simulink model "xz2dof_traj"  (R2023a)
settings: Solver=ode4  StartTime=0.0  StopTime=50  FixedStep=0.0001  RelTol=1e-3
values from neighbouring files (symbols this model uses):
  B1 = inv(B)    [grasp_test.m]    (also in my_mpc.m = inv(B0); xz2dof_para.m)
  C1 = C    [grasp_test.m]    (also in xz2dof_para.m)
  g = 9.8    [grasp_test.m]    (also in my_mpc.m; track_test.m; xz2dof_para.m)
  hL1 = 0.001    [grasp_test.m]    (also in my_mpc.m; xz2dof_para.m)
  hL2 = 0.001    [grasp_test.m]    (also in my_mpc.m; xz2dof_para.m)
  Iyy = 3*0.114    (= 0.342)    [my_mpc.m]    (also in track_test.m; xz2dof_para.m)
  kdq1 = 800    [grasp_test.m]    (also in xz2dof_para.m)
  kdq2 = 300    [grasp_test.m]    (also in xz2dof_para.m)
  kdx = 0.8    [track_test.m]    (also in xz2dof_para.m = 17)
  kdz = 1.5    [track_test.m]    (also in xz2dof_para.m = 50)
  kiq1 = 500    [grasp_test.m]    (also in xz2dof_para.m)
  kiq2 = 1000    [grasp_test.m]    (also in xz2dof_para.m)
  kix = 0    [track_test.m]    (also in xz2dof_para.m = 10)
  kiz = 0    [track_test.m]    (also in xz2dof_para.m)
  kpq1 = 1200    [grasp_test.m]    (also in xz2dof_para.m)
  kpq2 = 2000    [grasp_test.m]    (also in xz2dof_para.m)
  kpx = 1    [track_test.m]    (also in xz2dof_para.m = 180)
  kpz = 1.8    [track_test.m]    (also in xz2dof_para.m = 50)
  ktd = 10    [grasp_test.m]    (also in xz2dof_para.m)
  ktp = 1    [grasp_test.m]    (also in xz2dof_para.m)
  L1 = 0.12    [grasp_test.m]    (also in my_mpc.m; xz2dof_para.m)
  L2 = 0.12    [grasp_test.m]    (also in my_mpc.m; xz2dof_para.m)
  mb = 1.58    [my_mpc.m]    (also in track_test.m = 1.8; xz2dof_para.m = 1.8)
  mL1 = 0.1    [my_mpc.m]    (also in track_test.m = 0.08; xz2dof_para.m = 0.08)
  mL2 = 0.1    [my_mpc.m]    (also in track_test.m = 0.08; xz2dof_para.m = 0.08)
  ms = mb+mL1+mL2    (= 1.78)    [my_mpc.m]    (also in track_test.m = 1.96; xz2dof_para.m = 1.96)
  q1 = pi/2    (= 1.57079632679)    [grasp_test.m]    (also in my_mpc.m = xd(4) + xe(4); xz2dof_para.m)
  q2 = 0    [grasp_test.m]    (also in my_mpc.m = xd(5) + xe(5); xz2dof_para.m)
  step_num = T/tstep    (= 100)    [grasp_test.m]
undefined symbols (not defined in the file or in its folder): arm_traj
libraries: dspindex x1
settings Model: Creator=Administrator  LastModifiedBy=User
settings SolverCC: AlgebraicLoopSolver=TrustRegion
settings DataIOCC: ReturnWorkspaceOutputs=off
settings DebuggingCC: UnconnectedInputMsg=warning  UnconnectedOutputMsg=warning  UnconnectedLineMsg=warning
settings ModelReferenceCC: EnableRefExpFcnMdlSchedulingChecks=on
settings SFSimCC: CustomCodeUndefinedFunction=UseInterfaceOnly

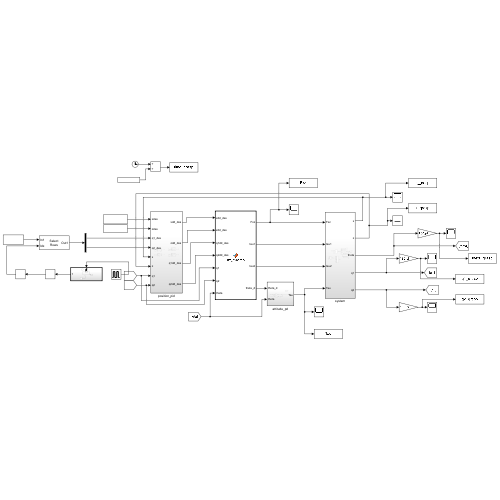
[thumbnail: Simulink's stored preview of the top-level diagram]
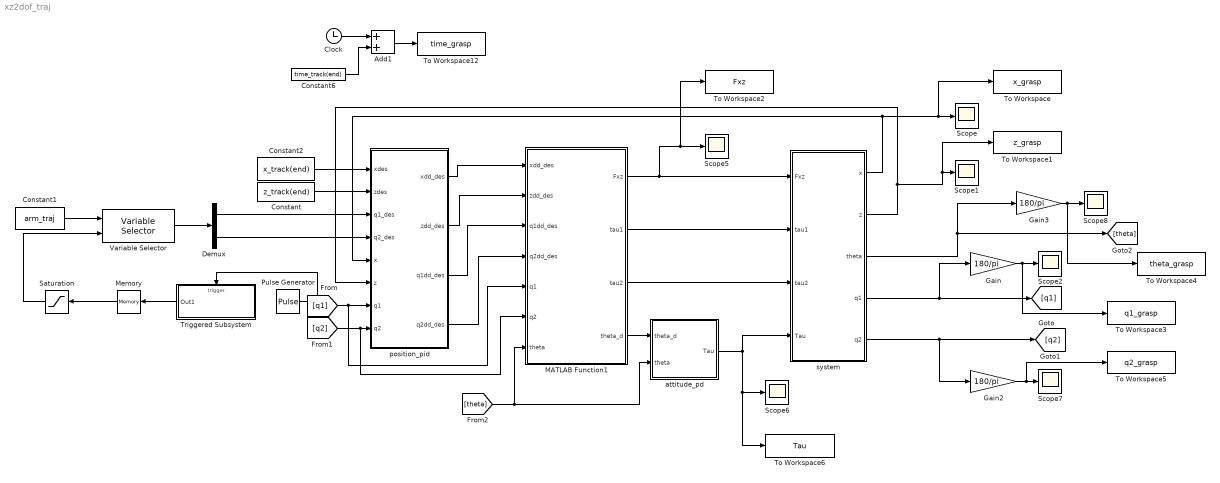
== system xz2dof_traj ==
  Add1 : Sum
  Clock : Clock
  Constant : Constant  Value=z_track(end)
  Constant1 : Constant  Value=arm_traj
  Constant2 : Constant  Value=x_track(end)
  Constant6 : Constant  Value=time_track(end)
  Demux : Demux  Outputs=2
  Gain : Gain  Gain=180/pi
  Gain2 : Gain  Gain=180/pi
  Gain3 : Gain  Gain=180/pi
  MATLAB Function1 : MATLAB Function  TreatAsAtomicUnit=on
  Memory : Memory
  Pulse Generator : DiscretePulseGenerator  PulseType=Time based  Period=0.5  PulseWidth=50
  Saturation : Saturate  UpperLimit=step_num  LowerLimit=0
  Scope{,1..2,5..8} (7 alike) : Scope
  To Workspace : ToWorkspace  VariableName=x_grasp  SampleTime=-1
  To Workspace1 : ToWorkspace  VariableName=z_grasp  SampleTime=-1
  To Workspace12 : ToWorkspace  VariableName=time_grasp  SampleTime=-1
  To Workspace2 : ToWorkspace  VariableName=Fxz  SampleTime=-1
  To Workspace3 : ToWorkspace  VariableName=q1_grasp  SampleTime=-1
  To Workspace4 : ToWorkspace  VariableName=theta_grasp  SampleTime=-1
  To Workspace5 : ToWorkspace  VariableName=q2_grasp  SampleTime=-1
  To Workspace6 : ToWorkspace  VariableName=Tau  SampleTime=-1
  Triggered Subsystem : Subsystem  TreatAsAtomicUnit=on
  Variable Selector : dspindex/Variable Selector  NumInputs=1  rowsOrCols=Rows  IdxMode=Variable  Elements=[1 3]  ZerOneIdxMode=Zero-based  errmode=Clip Index  FillMode=on  FillValues=0
  attitude_pd : Subsystem
  position_pid : Subsystem
  system : Subsystem
  wires:
  MATLAB Function1/4(theta_d) -> attitude_pd/1(theta_d)
  MATLAB Function1/1(Fxz) -> To Workspace2/1, Scope5/1, system/1(Fxz)
  attitude_pd/1(Tau) -> To Workspace6/1, Scope6/1, system/4(Tau)
  system/2(z) -> To Workspace1/1, Scope1/1, position_pid/6(z)
  system/1(x) -> To Workspace/1, Scope/1, position_pid/5(x)
  Gain/1 -> To Workspace3/1, Scope2/1
  Constant/1 -> position_pid/2(zdes)
  Constant2/1 -> position_pid/1(xdes)
  Add1/1 -> To Workspace12/1
  Clock/1 -> Add1/1
  Constant6/1 -> Add1/2
  [q1] -> MATLAB Function1/5(q1), position_pid/7(q1)
  system/5(q2) -> Gain2/1, [q2]
  Gain2/1 -> To Workspace5/1, Scope7/1
  [q2] -> MATLAB Function1/6(q2), position_pid/8(q2)
  position_pid/1(xdd_des) -> MATLAB Function1/1(xdd_des)
  position_pid/2(zdd_des) -> MATLAB Function1/2(zdd_des)
  position_pid/3(q1dd_des) -> MATLAB Function1/3(q1dd_des)
  position_pid/4(q2dd_des) -> MATLAB Function1/4(q2dd_des)
  MATLAB Function1/2(tau1) -> system/2(tau1)
  MATLAB Function1/3(tau2) -> system/3(tau2)
  Gain3/1 -> To Workspace4/1, Scope8/1
  system/3(theta) -> [theta], Gain3/1
  [theta] -> attitude_pd/2(theta), MATLAB Function1/7(theta)
  system/4(q1) -> Gain/1, [q1]
  Constant1/1 -> Variable Selector/1
  Variable Selector/1 -> Demux/1
  Memory/1 -> Saturation/1
  Triggered Subsystem/1(Out1) -> Memory/1
  Pulse Generator/1 -> Triggered Subsystem/Trigger
  Saturation/1 -> Variable Selector/2
  Demux/1 -> position_pid/3(q1_des)
  Demux/2 -> position_pid/4(q2_des)

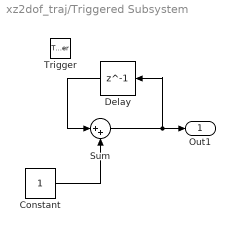
== system xz2dof_traj/Triggered Subsystem ==
  Trigger : TriggerPort  VariantControl=Variant
  Constant : Constant
  Delay : Delay  DelayLength=1
  Sum : Sum  Inputs=|++
  Out1 : Outport  VectorParamsAs1DForOutWhenUnconnected=off
  wires:
  Sum/1 -> Delay/1, Out1/1
  Constant/1 -> Sum/2
  Delay/1 -> Sum/1

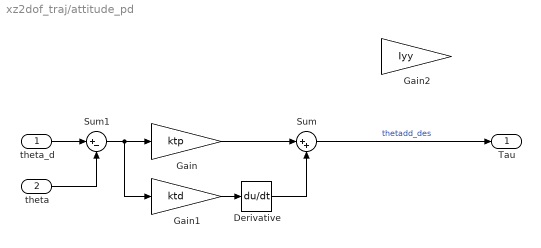
== system xz2dof_traj/attitude_pd ==
  theta_d : Inport
  theta : Inport  Port=2
  Derivative : Derivative
  Gain : Gain  Gain=ktp
  Gain1 : Gain  Gain=ktd
  Gain2 : Gain  Gain=Iyy
  Sum : Sum  Inputs=|++
  Sum1 : Sum  Inputs=|+-
  Tau : Outport  VectorParamsAs1DForOutWhenUnconnected=off
  wires:
  theta/1 -> Sum1/2
  Gain1/1 -> Derivative/1
  Derivative/1 -> Sum/2
  Sum1/1 -> Gain1/1, Gain/1
  Gain/1 -> Sum/1
  theta_d/1 -> Sum1/1
  Sum/1 -> Tau/1  "thetadd_des"

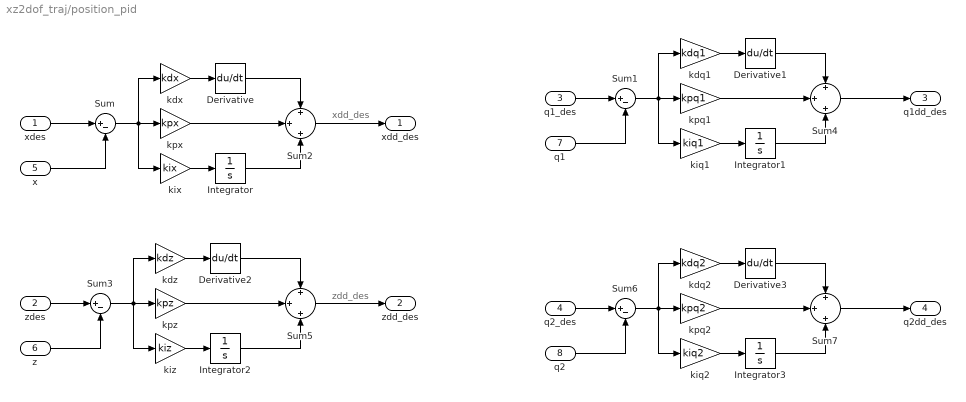
== system xz2dof_traj/position_pid ==
  note: zdd_des
  note: xdd_des
  xdes : Inport
  zdes : Inport  Port=2
  q1_des : Inport  Port=3
  q2_des : Inport  Port=4
  x : Inport  Port=5
  z : Inport  Port=6
  q1 : Inport  Port=7
  q2 : Inport  Port=8
  Derivative{,1..3} (4 alike) : Derivative
  Integrator{,1..3} (4 alike) : Integrator
  Sum{,1,3,6} (4 alike) : Sum  Inputs=|+-
  Sum{2,4..5,7} (4 alike) : Sum  Inputs=+|+|+
  kdq1 : Gain  Gain=kdq1
  kdq2 : Gain  Gain=kdq2
  kdx : Gain  Gain=kdx
  kdz : Gain  Gain=kdz
  kiq1 : Gain  Gain=kiq1
  kiq2 : Gain  Gain=kiq2
  kix : Gain  Gain=kix
  kiz : Gain  Gain=kiz
  kpq1 : Gain  Gain=kpq1
  kpq2 : Gain  Gain=kpq2
  kpx : Gain  Gain=kpx
  kpz : Gain  Gain=kpz
  xdd_des : Outport  VectorParamsAs1DForOutWhenUnconnected=off
  zdd_des : Outport  Port=2  VectorParamsAs1DForOutWhenUnconnected=off
  q1dd_des : Outport  Port=3  VectorParamsAs1DForOutWhenUnconnected=off
  q2dd_des : Outport  Port=4  VectorParamsAs1DForOutWhenUnconnected=off
  wires:
  kpz/1 -> Sum5/2
  kiz/1 -> Integrator2/1
  xdes/1 -> Sum/1
  kpx/1 -> Sum2/2
  z/1 -> Sum3/2
  Sum/1 -> kix/1, kpx/1, kdx/1
  kdx/1 -> Derivative/1
  Integrator/1 -> Sum2/3
  kdz/1 -> Derivative2/1
  Derivative/1 -> Sum2/1
  Derivative2/1 -> Sum5/1
  Sum3/1 -> kiz/1, kpz/1, kdz/1
  Integrator2/1 -> Sum5/3
  kix/1 -> Integrator/1
  x/1 -> Sum/2
  zdes/1 -> Sum3/1
  kpq1/1 -> Sum4/2
  kiq1/1 -> Integrator1/1
  Integrator1/1 -> Sum4/3
  kdq1/1 -> Derivative1/1
  Derivative1/1 -> Sum4/1
  Sum1/1 -> kiq1/1, kpq1/1, kdq1/1
  q1/1 -> Sum1/2
  q1_des/1 -> Sum1/1
  Sum2/1 -> xdd_des/1
  Sum5/1 -> zdd_des/1
  Sum4/1 -> q1dd_des/1
  Sum7/1 -> q2dd_des/1
  q2_des/1 -> Sum6/1
  Sum6/1 -> kiq2/1, kpq2/1, kdq2/1
  Derivative3/1 -> Sum7/1
  q2/1 -> Sum6/2
  kdq2/1 -> Derivative3/1
  Integrator3/1 -> Sum7/3
  kiq2/1 -> Integrator3/1
  kpq2/1 -> Sum7/2

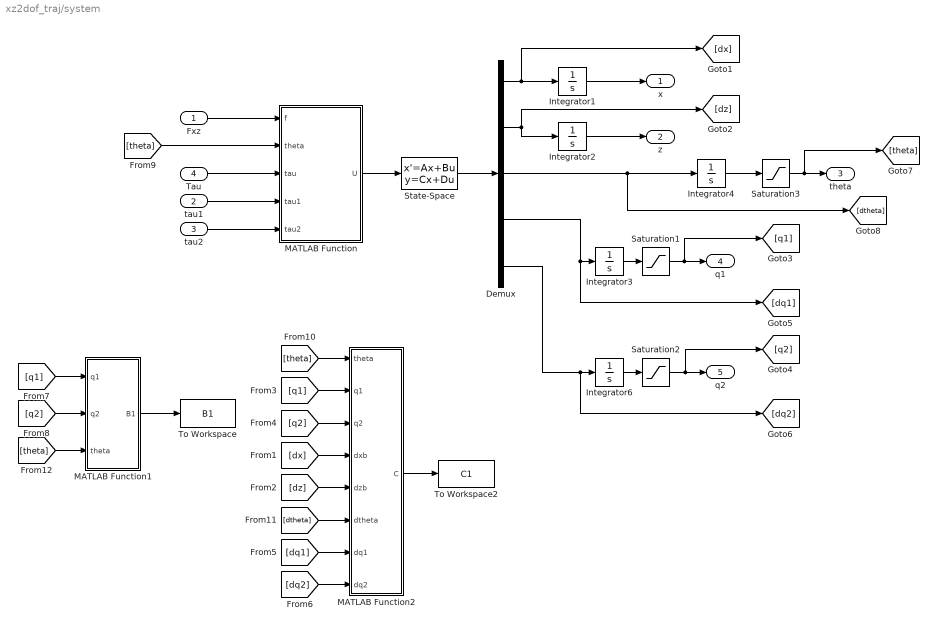
== system xz2dof_traj/system ==
  Fxz : Inport
  tau1 : Inport  Port=2
  tau2 : Inport  Port=3
  Tau : Inport  Port=4
  Demux : Demux  Outputs=5
  Integrator1 : Integrator  InitialCondition=x_track(end)
  Integrator2 : Integrator  InitialCondition=z_track(end)
  Integrator3 : Integrator  InitialCondition=pi/2
  Integrator4 : Integrator
  Integrator6 : Integrator
  MATLAB Function : MATLAB Function  TreatAsAtomicUnit=on
  MATLAB Function1 : MATLAB Function  TreatAsAtomicUnit=on
  MATLAB Function2 : MATLAB Function  TreatAsAtomicUnit=on
  Saturation1 : Saturate  UpperLimit=pi  LowerLimit=-pi
  Saturation2 : Saturate  UpperLimit=pi  LowerLimit=-pi
  Saturation3 : Saturate  UpperLimit=pi/2  LowerLimit=-pi/2
  State-Space : StateSpace  A=-B1*C1  B=B1  C=[1 0 0 0 0;0 1 0 0 0;0 0 1 0 0;0 0 0 1 0;0 0 0 0 1]  D=[0 0 0 0 0;0 0 0 0 0;0 0 0 0 0;0 0 0 0 0;0 0 0 0 0]  InitialCondition=0
  To Workspace : ToWorkspace  VariableName=B1  SaveFormat=Timeseries  SampleTime=-1
  To Workspace2 : ToWorkspace  VariableName=C1  SaveFormat=Timeseries  SampleTime=-1
  x : Outport  VectorParamsAs1DForOutWhenUnconnected=off
  z : Outport  Port=2  VectorParamsAs1DForOutWhenUnconnected=off
  theta : Outport  Port=3  VectorParamsAs1DForOutWhenUnconnected=off
  q1 : Outport  Port=4  VectorParamsAs1DForOutWhenUnconnected=off
  q2 : Outport  Port=5  VectorParamsAs1DForOutWhenUnconnected=off
  wires:
  Fxz/1 -> MATLAB Function/1(f)
  tau1/1 -> MATLAB Function/4(tau1)
  MATLAB Function/1(U) -> State-Space/1
  MATLAB Function1/1(B1) -> To Workspace/1
  State-Space/1 -> Demux/1
  Demux/1 -> [dx], Integrator1/1
  Demux/2 -> [dz], Integrator2/1
  Integrator1/1 -> x/1
  Integrator2/1 -> z/1
  Integrator3/1 -> Saturation1/1
  Demux/4 -> [dq1], Integrator3/1
  Saturation1/1 -> [q1], q1/1
  Saturation2/1 -> q2/1, [q2]
  Integrator6/1 -> Saturation2/1
  Demux/5 -> Integrator6/1, [dq2]
  [dx] -> MATLAB Function2/4(dxb)
  [dz] -> MATLAB Function2/5(dzb)
  [q1] -> MATLAB Function2/2(q1)
  [q2] -> MATLAB Function2/3(q2)
  [dq1] -> MATLAB Function2/7(dq1)
  [dq2] -> MATLAB Function2/8(dq2)
  [q1] -> MATLAB Function1/1(q1)
  [q2] -> MATLAB Function1/2(q2)
  [theta] -> MATLAB Function/2(theta)
  [theta] -> MATLAB Function2/1(theta)
  [dtheta] -> MATLAB Function2/6(dtheta)
  [theta] -> MATLAB Function1/3(theta)
  tau2/1 -> MATLAB Function/5(tau2)
  Tau/1 -> MATLAB Function/3(tau)
  Saturation3/1 -> [theta], theta/1
  Integrator4/1 -> Saturation3/1
  Demux/3 -> [dtheta], Integrator4/1
  MATLAB Function2/1(C) -> To Workspace2/1

== matlab function xz2dof_traj/system/MATLAB Function1 ==
  data: q1 input; q2 input; theta input; B1 output; mL1 parameter; mL2 parameter; mb parameter; L1 parameter; L2 parameter; hL1 parameter; hL2 parameter; Iyy parameter
function B1 = Bout(q1, q2, theta, mL1, mL2, mb, L1, L2, hL1, hL2, Iyy)
B = zeros(5,5);

B(1,1) = mL1 + mL2 + mb; B(1,2) = 0;
B(1,3) = (mL1*L1/2 + mL2*L1)*sin(q1-theta) + (mL2*L2/2)*sin(q1+q2-theta);
B(1,4) = -(mL1*L1/2 + mL2*L1)*sin(q1-theta) - (mL2*L2/2)*sin(q1+q2-theta);
B(1,5) = -(mL2*L2/2)*sin(q1+q2-theta);

B(2,1) = 0; B(2,2) = mL1 + mL2 + mb;
B(2,3) = -(mL1*L1/2 + mL2*L1)*cos(q1-theta) - (mL2*L2/2)*cos(q1+q2-theta);
B(2,4) = (mL1*L1/2 + mL2*L1)*cos(q1-theta) + (mL2*L2/2)*cos(q1+q2-theta);
B(2,5) = (mL2*L2/2)*cos(q1+q2-theta);

B(3,1) = (mL1*L1/2 + mL2*L1)*sin(q1-theta) + (mL2*L2/2)*sin(q1+q2-theta);
B(3,2) = -(mL1*L1/2 + mL2*L1)*cos(q1-theta) - (mL2*L2/2)*cos(q1+q2-theta);
B(3,3) = hL1 + hL2 + Iyy + mL1*(L1/2)^2 + mL2*(L1^2 + (L2/2)^2 + L1*L2*cos(q2)); 
B(3,4) = -mL2*(L1^2 + (L2/2)^2 + L1*L2*cos(q2)) - mL1*(L1/2)^2;
B(3,5) = -mL2*L2/2*(L2/2+L1*cos(q2));

B(4,1) = -(mL1*L1/2 + mL2*L1)*sin(q1-theta) - (mL2*L2/2)*sin(q1+q2-theta);
B(4,2) = (mL1*L1/2 + mL2*L1)*cos(q1-theta) + (mL2*L2/2)*cos(q1+q2-theta);
B(4,3) = -mL2*(L1^2 + (L2/2)^2 + L1*L2*cos(q2)) - mL1*(L1/2)^2;
B(4,4) = mL1*(L1/2)^2 + mL2*(L1^2 + (L2/2)^2 + L1*L2*cos(q2));
B(4,5) = mL2*L2/2*(L1*cos(q2) + L2/2);

B(5,1) = -(mL2*L2/2)*sin(q1+q2-theta);
B(5,2) = (mL2*L2/2)*cos(q1+q2-theta);
B(5,3) = -mL2*L2/2*(L2/2+L1*cos(q2));
B(5,4) = mL2*L2/2*(L1*cos(q2) + L2/2);
B(5,5) = mL2*L2*L2/4;

B1 = inv(B);

end

== matlab function xz2dof_traj/system/MATLAB Function ==
  data: f input; theta input; tau input; tau1 input; U output; tau2 input; q1 parameter; q2 parameter; g parameter; mL1 parameter; mL2 parameter; mb parameter; L1 parameter; L2 parameter
function U = Uout(f,theta,tau,tau1,tau2,q1,q2,g, mL1, mL2, mb, L1, L2)
u = zeros(5,1);
G = zeros(5,1);
U = zeros(5,1);

% f = f1+f2+f3+f4 是总升力
% tau是俯仰力矩
% tau1,tau2是关节力矩
u(1,1) = f*sin(theta);
u(2,1) = f*cos(theta);
u(3,1) = tau;
u(4,1) = tau1;
u(5,1) = tau2;

%% 计算G
G(1,1) = 0;
G(2,1) = (mL1 + mL2 + mb)*g;
G(3,1) = - g*mL1*(L1/2*cos(q1-theta)) - g*mL2*(L1*cos(q1-theta)+L2/2*cos(q1+q2-theta));
G(4,1) = g*mL1*(L1/2*cos(q1-theta)) + g*mL2*(L1*cos(q1-theta)+L2/2*cos(q1+q2-theta));
G(5,1) = g*mL2*L2/2*cos(q1 + q2-theta);

U = u - G;
end

== matlab function xz2dof_traj/system/MATLAB Function2 ==
  data: theta input; C output; q1 input; q2 input; dxb input; dzb input; dtheta input; dq1 input; dq2 input; mL1 parameter; mL2 parameter; L1 parameter; L2 parameter
function C = Cout(theta, q1, q2, dxb, dzb, dtheta, dq1, dq2, mL1, mL2, L1, L2)
C = zeros(5,5);

C(1,1) = 0; C(1,2) = 0;
C(1,3) =  dq1*(cos(q1 - theta)*((L1*mL1)/2 + L1*mL2) + (L2*mL2*cos(q1 + q2 - theta))/2) - dtheta*(cos(q1 - theta)*((L1*mL1)/2 + L1*mL2) + (L2*mL2*cos(q1 + q2 - theta))/2) + (L2*dq2*mL2*cos(q1 + q2 - theta))/2;
C(1,4) = dtheta*(cos(q1 - theta)*((L1*mL1)/2 + L1*mL2) + (L2*mL2*cos(q1 + q2 - theta))/2) - dq1*(cos(q1 - theta)*((L1*mL1)/2 + L1*mL2) + (L2*mL2*cos(q1 + q2 - theta))/2) - (L2*dq2*mL2*cos(q1 + q2 - theta))/2;
C(1,5) = (L2*dtheta*mL2*cos(q1 + q2 - theta))/2 - (L2*dq2*mL2*cos(q1 + q2 - theta))/2 - (L2*dq1*mL2*cos(q1 + q2 - theta))/2;

C(2,1) = 0; C(2,2) = 0;
C(2,3) = dq1*(sin(q1 - theta)*((L1*mL1)/2 + L1*mL2) + (L2*mL2*sin(q1 + q2 - theta))/2) - dtheta*(sin(q1 - theta)*((L1*mL1)/2 + L1*mL2) + (L2*mL2*sin(q1 + q2 - theta))/2) + (L2*dq2*mL2*sin(q1 + q2 - theta))/2;
C(2,4) = dtheta*(sin(q1 - theta)*((L1*mL1)/2 + L1*mL2) + (L2*mL2*sin(q1 + q2 - theta))/2) - dq1*(sin(q1 - theta)*((L1*mL1)/2 + L1*mL2) + (L2*mL2*sin(q1 + q2 - theta))/2) - (L2*dq2*mL2*sin(q1 + q2 - theta))/2;
C(2,5) = (L2*dtheta*mL2*sin(q1 + q2 - theta))/2 - (L2*dq2*mL2*sin(q1 + q2 - theta))/2 - (L2*dq1*mL2*sin(q1 + q2 - theta))/2;
 
C(3,1) = dq1*(cos(q1 - theta)*((L1*mL1)/2 + L1*mL2) + (L2*mL2*cos(q1 + q2 - theta))/2) - dtheta*(cos(q1 - theta)*((L1*mL1)/2 + L1*mL2) + (L2*mL2*cos(q1 + q2 - theta))/2) + (L2*dq2*mL2*cos(q1 + q2 - theta))/2;
C(3,2) = dq1*(sin(q1 - theta)*((L1*mL1)/2 + L1*mL2) + (L2*mL2*sin(q1 + q2 - theta))/2) - dtheta*(sin(q1 - theta)*((L1*mL1)/2 + L1*mL2) + (L2*mL2*sin(q1 + q2 - theta))/2) + (L2*dq2*mL2*sin(q1 + q2 - theta))/2;
C(3,3) = - dxb*(cos(q1 - theta)*((L1*mL1)/2 + L1*mL2) + (L2*mL2*cos(q1 + q2 - theta))/2) - dzb*(sin(q1 - theta)*((L1*mL1)/2 + L1*mL2) + (L2*mL2*sin(q1 + q2 - theta))/2) - (L1*L2*dq2*mL2*sin(q2))/2;
C(3,4) = dxb*(cos(q1 - theta)*((L1*mL1)/2 + L1*mL2) + (L2*mL2*cos(q1 + q2 - theta))/2) + dzb*(sin(q1 - theta)*((L1*mL1)/2 + L1*mL2) + (L2*mL2*sin(q1 + q2 - theta))/2) + (L1*L2*dq2*mL2*sin(q2))/2;
C(3,5) = (L2*dzb*mL2*sin(q1 + q2 - theta))/2 + (L2*dxb*mL2*cos(q1 + q2 - theta))/2 + (L1*L2*dq1*mL2*sin(q2))/2 + (L1*L2*dq2*mL2*sin(q2))/2 - (L1*L2*dtheta*mL2*sin(q2))/2;

C(4,1) = dtheta*(cos(q1 - theta)*((L1*mL1)/2 + L1*mL2) + (L2*mL2*cos(q1 + q2 - theta))/2) - dq1*(cos(q1 - theta)*((L1*mL1)/2 + L1*mL2) + (L2*mL2*cos(q1 + q2 - theta))/2) - (L2*dq2*mL2*cos(q1 + q2 - theta))/2;
C(4,2) = dtheta*(sin(q1 - theta)*((L1*mL1)/2 + L1*mL2) + (L2*mL2*sin(q1 + q2 - theta))/2) - dq1*(sin(q1 - theta)*((L1*mL1)/2 + L1*mL2) + (L2*mL2*sin(q1 + q2 - theta))/2) - (L2*dq2*mL2*sin(q1 + q2 - theta))/2;
C(4,3) = dxb*(cos(q1 - theta)*((L1*mL1)/2 + L1*mL2) + (L2*mL2*cos(q1 + q2 - theta))/2) + dzb*(sin(q1 - theta)*((L1*mL1)/2 + L1*mL2) + (L2*mL2*sin(q1 + q2 - theta))/2) + (L1*L2*dq2*mL2*sin(q2))/2;
C(4,4) = - dxb*(cos(q1 - theta)*((L1*mL1)/2 + L1*mL2) + (L2*mL2*cos(q1 + q2 - theta))/2) - dzb*(sin(q1 - theta)*((L1*mL1)/2 + L1*mL2) + (L2*mL2*sin(q1 + q2 - theta))/2) - (L1*L2*dq2*mL2*sin(q2))/2;
C(4,5) = (L1*L2*dtheta*mL2*sin(q2))/2 - (L2*dxb*mL2*cos(q1 + q2 - theta))/2 - (L1*L2*dq1*mL2*sin(q2))/2 - (L1*L2*dq2*mL2*sin(q2))/2 - (L2*dzb*mL2*sin(q1 + q2 - theta))/2;

C(5,1) = (L2*dtheta*mL2*cos(q1 + q2 - theta))/2 - (L2*dq2*mL2*cos(q1 + q2 - theta))/2 - (L2*dq1*mL2*cos(q1 + q2 - theta))/2;
C(5,2) = (L2*dtheta*mL2*sin(q1 + q2 - theta))/2 - (L2*dq2*mL2*sin(q1 + q2 - theta))/2 - (L2*dq1*mL2*sin(q1 + q2 - theta))/2;
C(5,3) = (L2*dzb*mL2*sin(q1 + q2 - theta))/2 + (L2*dxb*mL2*cos(q1 + q2 - theta))/2 + (L1*L2*dq1*mL2*sin(q2))/2 + (L1*L2*dq2*mL2*sin(q2))/2 - (L1*L2*dtheta*mL2*sin(q2))/2;
C(5,4) = (L1*L2*dtheta*mL2*sin(q2))/2 - (L2*dxb*mL2*cos(q1 + q2 - theta))/2 - (L1*L2*dq1*mL2*sin(q2))/2 - (L1*L2*dq2*mL2*sin(q2))/2 - (L2*dzb*mL2*sin(q1 + q2 - theta))/2;
C(5,5) = (L1*L2*dtheta*mL2*sin(q2))/2 - (L2*dxb*mL2*cos(q1 + q2 - theta))/2 - (L1*L2*dq1*mL2*sin(q2))/2 - (L2*dzb*mL2*sin(q1 + q2 - theta))/2;


end

== matlab function xz2dof_traj/MATLAB Function1 ==
  data: xdd_des input; Fxz output; tau1 output; tau2 output; zdd_des input; q1dd_des input; q2dd_des input; q1 input; q2 input; theta input; theta_d output; ms parameter; g parameter; hL1 parameter; mL1 parameter; L1 parameter; mL2 parameter; L2 parameter; hL2 parameter
function [Fxz,tau1,tau2,theta_d] = inv_dynamic(xdd_des, zdd_des, q1dd_des, q2dd_des, q1, q2, theta, ms, g, hL1, mL1, L1, mL2, L2, hL2)
Fxz = ms*sqrt((xdd_des)^2+(zdd_des+g)^2);
theta_d = atan(xdd_des/(zdd_des+g));
tau1 = hL1*q1dd_des - mL1*g*L1/2*cos(q1-theta) - mL2*g*(L1*cos(q1-theta)+L2/2*cos(q1+q2-theta));
tau2 = hL2*q2dd_des - mL2*g*L2/2*cos(q1+q2-theta);
end
